simulink model "testing"  (R2023b)
settings: Solver=VariableStepAuto  StartTime=0.0  StopTime=10.0  RelTol=1e-3
undefined symbols (not defined in the file): Ion, Lithium
libraries: spsACVoltageSourceLib x3, spsGroundLib x3, spsBatteryLib x1, spsPermanentMagnetSynchronousMachineLib x1, spsTriangleGeneratorLib x1
settings Model: Creator=bbassett6  LastModifiedBy=bbassett6

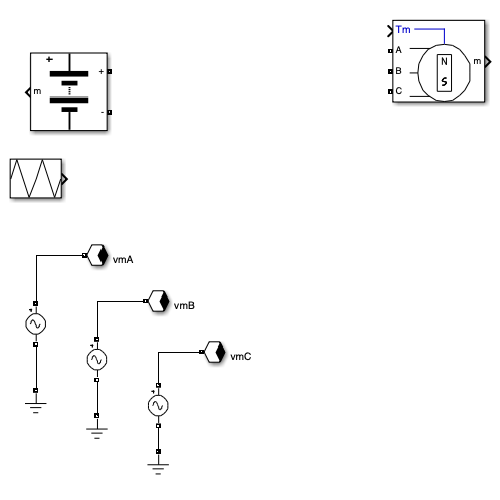
[thumbnail: Simulink's stored preview of the top-level diagram]
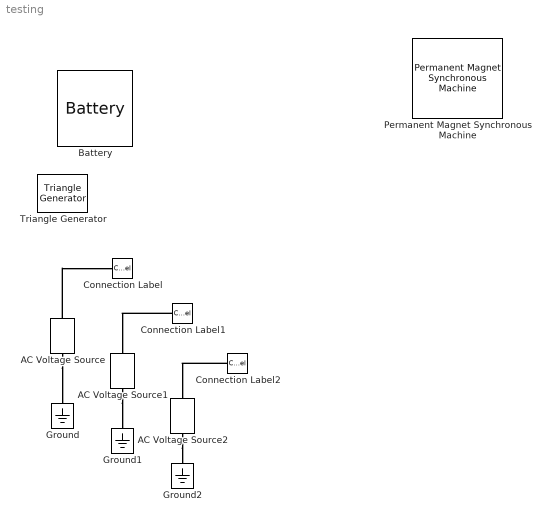
== system testing ==
  AC Voltage Source : spsACVoltageSourceLib/AC Voltage Source  Amplitude=5  Phase=0  Frequency=1e3  SampleTime=0  Measurements=None  BusType=swing  Pref=10e3  Qref=0  Qmin=-inf  Qmax=+inf
  AC Voltage Source1 : spsACVoltageSourceLib/AC Voltage Source  Amplitude=5  Phase=120  Frequency=60  SampleTime=0  Measurements=None  BusType=swing  Pref=10e3  Qref=0  Qmin=-inf  Qmax=+inf
  AC Voltage Source2 : spsACVoltageSourceLib/AC Voltage Source  Amplitude=5  Phase=240  Frequency=60  SampleTime=0  Measurements=None  BusType=swing  Pref=10e3  Qref=0  Qmin=-inf  Qmax=+inf
  Battery : spsBatteryLib/Battery  BatType=Lithium-Ion  ShowTempParam=off  ThermalPreset=no  ShowAgeParam=off  NomV=7.2  NomQ=5.4  SOC=100  Batt_Tr=30  PresetModel=on  MaxQ=5.4  MinV=5.4  FullV=8.3807  Dis_rate=2.3478  R=0.013333  Normal_OP=4.8835  expZone="[7.7788      0.2653]"  current=[6.5 13 32.5]  Units=Time  Tci=20  NomT=20  T2=-30  MaxQ2=4.8  FullV2=7.1  Normal_OP2=5.655  expZone2="[6.58           1]"  Rca=0.6  ti=2000  Dp=0  Neq0=0  Tsim=1e6  Ta1=25  Qeol=5.4*0.9  Reol=0.013333*1.2  Char_age=[2.3478, 3]  Dis_age=[2.3478, 10]  N1=1500  N2=10500  N3=1000  N4=1400  Ta2=45  N5=950
  Connection Label : ConnectionLabel  Label=vmA
  Connection Label1 : ConnectionLabel  Label=vmB
  Connection Label2 : ConnectionLabel  Label=vmC
  Ground : spsGroundLib/Ground  LConnTagsString=a
  Ground1 : spsGroundLib/Ground  LConnTagsString=a
  Ground2 : spsGroundLib/Ground  LConnTagsString=a
  Permanent Magnet Synchronous Machine : spsPermanentMagnetSynchronousMachineLib/Permanent Magnet Synchronous Machine  NbPhases=3  FluxDistribution=Sinusoidal  RotorType=Round  MechanicalLoad=Torque Tm  PresetModel="13:  42.09 Nm 560 Vdc 3000 RPM - 45.6 Nm"  ShowDetailedParameters=on  MeasurementBus=off  Resistance=0.0485  Inductance=8.5e-3  dqInductances=[8.5e-3,8.5e-3]  La=0.000395  MachineConstant=Flux linkage established by magnets (V.s)  Flux=0.1194  VoltageCst=86.6271  TorqueCst=0.7164  Flat=120  Mechanical=[0.0027 0.0004924 4 0]  PolePairs=4  InitialConditions=[0,0, 0,0]  InitialConditions5ph=[0 0 0 0 0 0]  RefAngle=90 degrees behind phase A axis (modified Park)  IterativeDiscreteModel=Trapezoidal non iterative  TsBlock=-1  TsPowergui=0
  Triangle Generator : spsTriangleGeneratorLib/Triangle Generator  Freq=1e5  Phase=90  Ts=0
  connections:
  AC Voltage Source/RConn1 -- Connection Label/LConn1
  AC Voltage Source/LConn1 -- Ground/LConn1
  AC Voltage Source1/LConn1 -- Ground1/LConn1
  AC Voltage Source2/LConn1 -- Ground2/LConn1
  Connection Label1/LConn1 -- AC Voltage Source1/RConn1
  Connection Label2/LConn1 -- AC Voltage Source2/RConn1
